simulink library "stateMachineHandler"  (R2016b)
settings: Solver=VariableStepAuto  StartTime=0.0  StopTime=10.0  RelTol=1e-3
settings Model: Creator=Nathan  LastModifiedBy=Taeke

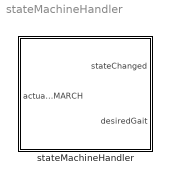
== system stateMachineHandler ==
  stateMachineHandler : Subsystem

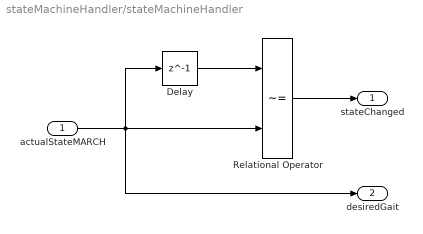
== system stateMachineHandler/stateMachineHandler ==
  actualStateMARCH : Inport
  Delay : Delay  DelayLength=1  InitialCondition=0
  Relational Operator : RelationalOperator  Operator=~=  OutDataTypeStr=boolean  RndMeth=Simplest
  stateChanged : Outport  BusOutputAsStruct=on
  desiredGait : Outport  Port=2
  wires:
  actualStateMARCH/1 -> Delay/1, Relational Operator/2, desiredGait/1
  Delay/1 -> Relational Operator/1
  Relational Operator/1 -> stateChanged/1
